simulink model "Peregrine_Falcon_Lab"  (R2024b)
settings: Solver=VariableStepAuto  StartTime=0.0  StopTime=10.0  RelTol=1e-3
undefined symbols (not defined in the file): A1, A2, Cd1, Cd2, g, m, rho
settings Model: Creator=Labden  LastModifiedBy=Labden

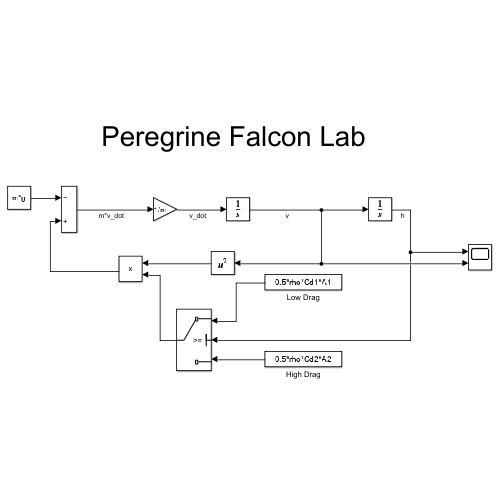
[thumbnail: Simulink's stored preview of the top-level diagram]
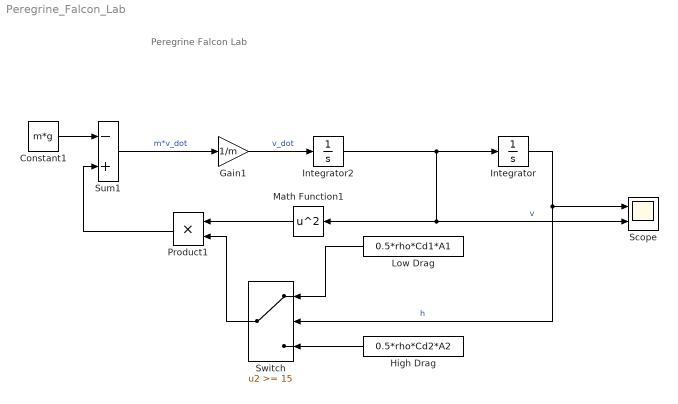
== system Peregrine_Falcon_Lab ==
  note: Peregrine Falcon Lab
  Constant1 : Constant  Value=m*g
  Gain1 : Gain  Gain=1/m
  High Drag : Constant  Value=0.5*rho*Cd2*A2
  Integrator : Integrator  InitialCondition=60
  Integrator2 : Integrator  InitialCondition=-10
  Low Drag : Constant  Value=0.5*rho*Cd1*A1
  Math Function1 : Math  Operator=square  SignedPower=on
  Product1 : Product
  Scope : Scope  NumInputPorts=2
  Sum1 : Sum  Inputs=-+
  Switch : Switch  Threshold=15  SaturateOnIntegerOverflow=off  InputSameDT=off
  wires:
  Switch/1 -> Product1/2
  Low Drag/1 -> Switch/1
  High Drag/1 -> Switch/3
  Math Function1/1 -> Product1/1
  Sum1/1 -> Gain1/1  "m*v_dot"
  Gain1/1 -> Integrator2/1  "v_dot"
  Constant1/1 -> Sum1/1
  Product1/1 -> Sum1/2
  Integrator/1 -> Switch/2, Scope/1  "h"
  Integrator2/1 -> Math Function1/1, Scope/2, Integrator/1  "v"
